simulink library "branch_library"  (R2021b)
settings: Solver=VariableStepAuto  StartTime=0.0  StopTime=10.0  RelTol=1e-3
libraries: spsThreePhaseSeriesRLCBranchLib x5
settings Model: Creator=lpwoolcock  LastModifiedBy=lpwoolcock
settings SolverCC: AlgebraicLoopSolver=TrustRegion
settings DebuggingCC: SFMachineParentedDataDiag=warning

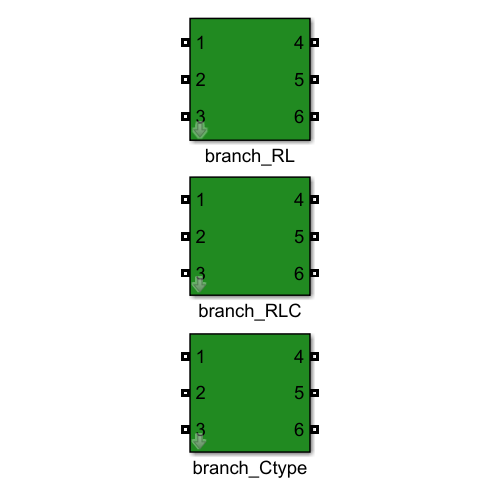
[thumbnail: Simulink's stored preview of the top-level diagram]
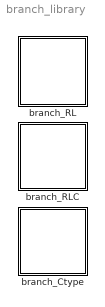
== system branch_library ==
  branch_Ctype : Subsystem  mask{C1=0, L=0, C=0, R=0}
      mask Display: patch([0 1 1 0], [0 0 1 1], [0.13 0.54 0.13])
  branch_RL : Subsystem  mask{R=0, L=0}
      mask prompts: R "Resistance"; L "Inductance"
      mask Display: patch([0 1 1 0], [0 0 1 1], [0.13 0.54 0.13])
  branch_RLC : Subsystem  mask{R=0, L=0, C=0}
      mask prompts: R "Resistance:"; L "Inductance:"; C "Capacitance:"
      mask Display: patch([0 1 1 0], [0 0 1 1], [0.13 0.54 0.13])

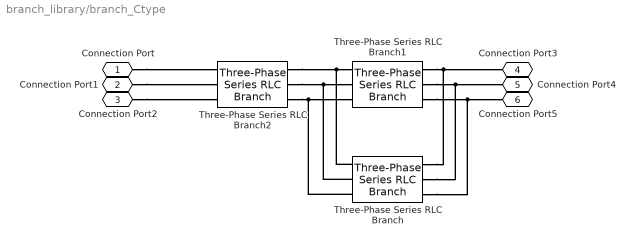
== system branch_library/branch_Ctype ==
  Three-Phase Series RLC Branch : spsThreePhaseSeriesRLCBranchLib/Three-Phase Series RLC Branch  LConnTagsString=A|B|C  RConnTagsString=A|B|C  BranchType=R  Resistance=R  Inductance=1e-3  Capacitance=1e-6  Measurements=None
  Three-Phase Series RLC Branch1 : spsThreePhaseSeriesRLCBranchLib/Three-Phase Series RLC Branch  LConnTagsString=A|B|C  RConnTagsString=A|B|C  BranchType=LC  Resistance=1  Inductance=L  Capacitance=C  Measurements=None
  Three-Phase Series RLC Branch2 : spsThreePhaseSeriesRLCBranchLib/Three-Phase Series RLC Branch  LConnTagsString=A|B|C  RConnTagsString=A|B|C  BranchType=C  Resistance=1  Inductance=1e-3  Capacitance=C1  Measurements=None
  Connection Port : PMIOPort  Side=Left
  Connection Port1 : PMIOPort  Port=2  Side=Left
  Connection Port2 : PMIOPort  Port=3  Side=Left
  Connection Port3 : PMIOPort  Port=4  Side=Right
  Connection Port4 : PMIOPort  Port=5  Side=Right
  Connection Port5 : PMIOPort  Port=6  Side=Right
  connections:
  Three-Phase Series RLC Branch1/RConn3 -- Three-Phase Series RLC Branch/RConn3 -- Connection Port5/RConn1
  Connection Port/RConn1 -- Three-Phase Series RLC Branch2/LConn1
  Three-Phase Series RLC Branch2/RConn3 -- Three-Phase Series RLC Branch/LConn3 -- Three-Phase Series RLC Branch1/LConn3
  Three-Phase Series RLC Branch2/RConn2 -- Three-Phase Series RLC Branch/LConn2 -- Three-Phase Series RLC Branch1/LConn2
  Three-Phase Series RLC Branch2/RConn1 -- Three-Phase Series RLC Branch/LConn1 -- Three-Phase Series RLC Branch1/LConn1
  Three-Phase Series RLC Branch1/RConn1 -- Three-Phase Series RLC Branch/RConn1 -- Connection Port3/RConn1
  Connection Port2/RConn1 -- Three-Phase Series RLC Branch2/LConn3
  Connection Port1/RConn1 -- Three-Phase Series RLC Branch2/LConn2
  Three-Phase Series RLC Branch1/RConn2 -- Three-Phase Series RLC Branch/RConn2 -- Connection Port4/RConn1

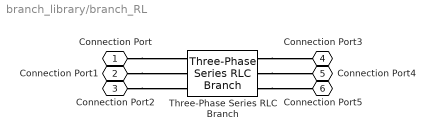
== system branch_library/branch_RL ==
  Three-Phase Series RLC Branch : spsThreePhaseSeriesRLCBranchLib/Three-Phase Series RLC Branch  LConnTagsString=A|B|C  RConnTagsString=A|B|C  BranchType=RL  Resistance=R  Inductance=L  Capacitance=1e-6  Measurements=None
  Connection Port : PMIOPort  Tag=PMCPort  Side=Left
  Connection Port1 : PMIOPort  Tag=PMCPort  Port=2  Side=Left
  Connection Port2 : PMIOPort  Tag=PMCPort  Port=3  Side=Left
  Connection Port3 : PMIOPort  Tag=PMCPort  Port=4  Side=Right
  Connection Port4 : PMIOPort  Tag=PMCPort  Port=5  Side=Right
  Connection Port5 : PMIOPort  Tag=PMCPort  Port=6  Side=Right
  connections:
  Three-Phase Series RLC Branch/RConn1 -- Connection Port3/RConn1
  Three-Phase Series RLC Branch/RConn3 -- Connection Port5/RConn1
  Three-Phase Series RLC Branch/RConn2 -- Connection Port4/RConn1
  Connection Port/RConn1 -- Three-Phase Series RLC Branch/LConn1
  Connection Port2/RConn1 -- Three-Phase Series RLC Branch/LConn3
  Connection Port1/RConn1 -- Three-Phase Series RLC Branch/LConn2

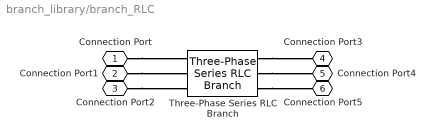
== system branch_library/branch_RLC ==
  Three-Phase Series RLC Branch : spsThreePhaseSeriesRLCBranchLib/Three-Phase Series RLC Branch  LConnTagsString=A|B|C  RConnTagsString=A|B|C  BranchType=RLC  Resistance=R  Inductance=L  Capacitance=C  Measurements=None
  Connection Port : PMIOPort  Tag=PMCPort  Side=Left
  Connection Port1 : PMIOPort  Tag=PMCPort  Port=2  Side=Left
  Connection Port2 : PMIOPort  Tag=PMCPort  Port=3  Side=Left
  Connection Port3 : PMIOPort  Tag=PMCPort  Port=4  Side=Right
  Connection Port4 : PMIOPort  Tag=PMCPort  Port=5  Side=Right
  Connection Port5 : PMIOPort  Tag=PMCPort  Port=6  Side=Right
  connections:
  Three-Phase Series RLC Branch/RConn2 -- Connection Port4/RConn1
  Three-Phase Series RLC Branch/RConn3 -- Connection Port5/RConn1
  Connection Port/RConn1 -- Three-Phase Series RLC Branch/LConn1
  Connection Port2/RConn1 -- Three-Phase Series RLC Branch/LConn3
  Three-Phase Series RLC Branch/RConn1 -- Connection Port3/RConn1
  Connection Port1/RConn1 -- Three-Phase Series RLC Branch/LConn2
